simulink model "web_adc"  (Simulink 7.3)
settings: Solver=FixedStepDiscrete  SolverMode=SingleTasking  StartTime=0.0  StopTime=10.0  RelTol=1e-3
PreLoadFcn:
  | waijung.modelPreload; % Required for working with Waijung Blockset. Do not remove.
undefined symbols (not defined in the file): A0, A1, A2, A3, A7, B0, B1, B10, B11, B12, B13, C1, C2, C3, C4, C5, HSEOSC, Link, LQFP176, ST, STM32F417IG
libraries: simulink x4, waijung_webserver x3, stm32f4_io_lib x1, stm32f4_adc_lib x1, stm32f4_device_config_lib x1, amg_sqlite_dataserver x1
CloseFcn:
  | waijung.modelClose; % Required for working with Waijung Blockset. Do not remove.
settings Model: Creator=Krisada  LastModifiedBy=Krisada
settings OptimizationCC: OptimizeModelRefInitCode=on  LifeSpan=1
settings HardwareCC: ProdEndianess=LittleEndian  ProdHWDeviceType=ARM Compatible->Cortex - M4  TargetEndianess=LittleEndian  TargetHWDeviceType=ARM Compatible->Cortex - M4
settings RTWCC: SystemTargetFile=stm32f4.tlc  GenerateMakefile=off  TemplateMakefile=ert_default_tmf  Description=STM32F4 Target  ProcessScript=stm32f4_make_rtw_hook
settings CodeAppCC: IgnoreCustomStorageClasses=off
settings STFCustomTargetCC: ModelReferenceCompliant=off  CombineOutputUpdateFcns=on  ERTCustomFileBanners=on  SupportContinuousTime=off  SupportNonInlinedSFcns=off  SystemTargetFile=stm32f4.tlc
settings ERTTargetCC: MultiwordLength=2048  ModelReferenceCompliant=off  ParMdlRefBuildCompliant=off  CompOptLevelCompliant=off  ERTFirstTimeCompliant=off  ModelStepFunctionPrototypeControlCompliant=off  CPPClassGenCompliant=off  ExtModeMexFile=noextcomm  InlinedParameterPlacement=NonHierarchical  ERTSrcFileBannerTemplate=stm32f4_code_template.cgt  ERTHdrFileBannerTemplate=stm32f4_code_template.cgt  ERTDataSrcFileTemplate=stm32f4_code_template.cgt  ERTDataHdrFileTemplate=stm32f4_code_template.cgt  ERTCustomFileTemplate=stm32f4_file_process.tlc

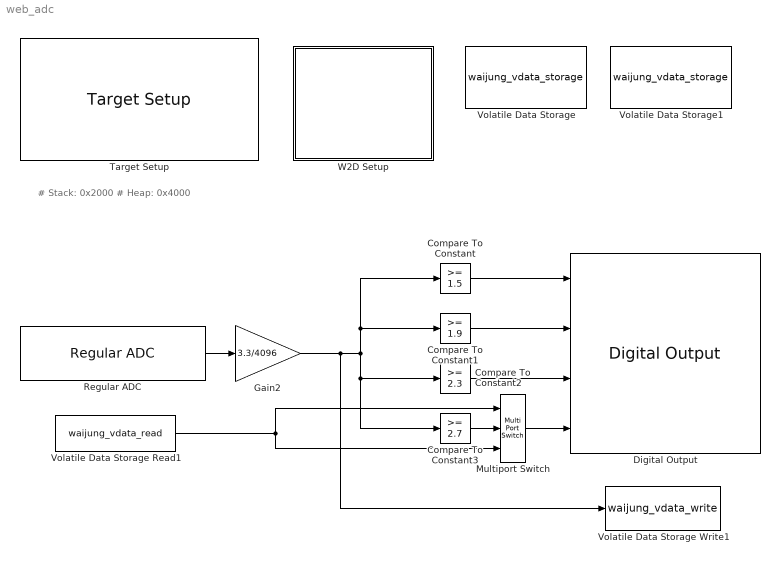
== system web_adc ==
  note: # Stack: 0x2000
      | # Heap: 0x4000
  Compare To Constant : simulink/Logic and Bit Operations/Compare To Constant  SystemSampleTime=-1  relop=>=  const=1.5  LogicOutDataTypeMode=uint8  ZeroCross=off
  Compare To Constant1 : simulink/Logic and Bit Operations/Compare To Constant  SystemSampleTime=-1  relop=>=  const=1.9  LogicOutDataTypeMode=uint8  ZeroCross=off
  Compare To Constant2 : simulink/Logic and Bit Operations/Compare To Constant  SystemSampleTime=-1  relop=>=  const=2.3  LogicOutDataTypeMode=uint8  ZeroCross=off
  Compare To Constant3 : simulink/Logic and Bit Operations/Compare To Constant  SystemSampleTime=-1  relop=>=  const=2.7  LogicOutDataTypeMode=uint8  ZeroCross=off
  Digital Output : stm32f4_io_lib/Digital Output  use_bitband=on  port=D  speed=100  porttype=Push Pull  porttypestr=PP  use_pin0=off  use_pin1=off  use_pin2=off  use_pin3=off  use_pin4=off  use_pin5=off  use_pin6=off  use_pin7=off  use_pin8=off  use_pin9=off  use_pin10=off  use_pin11=off  use_pin12=on  use_pin13=on  use_pin14=on  use_pin15=on  pinstr=GPIO_Pin_12 | GPIO_Pin_13 | GPIO_Pin_14 | GPIO_Pin_15  usedpinarray="[0  0  0  0  0  0  0  0  0  0  0  0  1  1  1  1]"  bitbandingstr=|  sampletime=-1  sampletimestr=0.01  blockid=DigitalOutput  enablecustomportlabel=off  globalinit=off  cinputportlabel=In1, In2  coutputportlabel=0
      | #define DigitalOutput_D12 Peripheral_BB(GPIOD->ODR, 12)  /* Output pin */
      | #define DigitalOutput_D13 Peripheral_BB(GPIOD->ODR, 13)  /* Output pin */
      | #define DigitalOutput_D14 Peripheral_BB(GPIOD->ODR, 14)  /* Output pin */
      | #define DigitalOutput_D15 Peripheral_BB(GPIOD->ODR, 15)  /* Output pin */
  Gain2 : Gain  Gain=3.3/4096  ParameterDataTypeMode=single  ParameterDataType=fixdt(1, 16)  ParameterScaling=2^0  ParamDataTypeStr=single  OutDataTypeMode=single  OutDataType=fixdt(1, 16)  OutScaling=2^0  OutDataTypeStr=single
  Multiport Switch : MultiPortSwitch  Inputs=2  zeroidx=on  OutDataType=fixdt(1, 16)  OutScaling=2^0
  Regular ADC : stm32f4_adc_lib/Regular ADC  adcmodule=1  outputdatatype=Double  prescaler=2  prescalerstr=ADC_Prescaler_Div2  chsamplingtime=Auto  chsamplingtimestr=ADC_SampleTime_480Cycles  read_an0=off  read_an1=off  read_an2=off  read_an3=off  read_an4=off  read_an5=off  read_an6=off  read_an7=off  read_an8=off  read_an9=off  read_an10=on  read_an11=off  read_an12=off  read_an13=off  read_an14=off  read_an15=off  read_an16=off  read_an17=off  read_an18=off  pinstr=GPIO_Pin_10  usedpinarray="[0  0  0  0  0  0  0  0  0  0  1  0  0  0  0  0  0  0  0]"  usedportidarray=[2]  usedpinidarray=[0]  usedpinidcount=1  sampletime=.01  blockid=RegularADC  enablecustomportlabel=off  cinputportlabel=0  coutputportlabel=Out1, Out2
  Target Setup : stm32f4_device_config_lib/Target Setup  Priority=100  compiler=GNU ARM  previous_compiler=GNU ARM  mcu=STM32F417IG (LQFP176)  mcustr=STM32F417IG  clockconfig=HSEOSC-8MHz  system_stm32f4xx_c_path=F:\trunk\targets\stm32f4_target\stm32f4\utils\system_stm32f4xx_default\STM32F40_41xxx\hseosc8mhz  showmemoryconfiguration=on  stacksize=0x2000  heapsize=0x4000  enableautocompiledownload=on  fullchiperase=off  programmerinterface=ST-Link  editctrlstr=on  compilercontrolstr=$(patsubst %, -I%, .) -mcpu=cortex-m4 -mthumb -mthumb-interwork -mfloat-abi=hard -mfpu=fpv4-sp-d16 -ffast-math -Wall -Wextra -Ofast  assemblercontrolstr=$(patsubst %, -I%, .) -mcpu=cortex-m4 -mthumb -mthumb-interwork -mfloat-abi=hard -mfpu=fpv4-sp-d16 -ffast-math -Wall -Wextra -Ofast -Wa,-amhls=$(<:.s=.lst) -D__STACK_SIZE=$(STACK_SIZE) -D__HEAP_SIZE=$(HEAP_SIZE)  linkercontrolstr=-T$(LD_SCRIPT) -g -Wl,-Map=$(MAP),--cref,--no-warn-mismatch -mcpu=cortex-m4 -mthumb -mthumb-interwork -mfloat-abi=hard -mfpu=fpv4-sp-d16 -specs=nosys.specs  runafterdownload=on  execprofile=None  profileruart=1  profilerbaud=115200  profilertxpin=D8  profilerinitstr=0.001,168000000,168000,115200,0  manualsetsampletime=off  sampletime=0.001  blockid=TargetSetup  systickreloadvalue=168000  hseval=8000000  lastprofileruart=1  hclk=168000000  flashorigin=0x8000000  flashlength=1024k  ramorigin=0x20000000  ramlength=128k  useextram=off
  Volatile Data Storage : S-Function  FunctionName=waijung_vdata_storage  Parameters=storagetype,storagename,initval,varname,buffersize,initvalstring,sampletime,sampletimestr,blockid,storagetypestr  EnableBusSupport=off  mask(waijung_vdata_storage){storagetype=single, storagename=adc, initval=0, varname=VolatileDataStorage_adc, buffersize=64, initvalstring='Initial string', webintegration=ReadOnly with KeyValuePair, weboutputformat='%f', webcgicallback=(void*)0, laststoragetype=single, sampletime=-1, sampletimestr=0.001, blockid=VolatileDataStorage, storagetypestr=float}
      mask prompts: storagetype "Storage Type"; storagename "Storage Name (must be a valid variable name)"; initval "Initial value (Apply at Power on Reset only)"; varname "Variable name"; buffersize "Size (bytes)"; initvalstring "Initial value (Apply at Power on Reset only)"; webintegration "Web CGI varget/varset integration"; weboutputformat "Web CGI varget output format"; webcgicallback "Web CGI varset callback"; laststoragetype "Last selected Storage Type"; sampletime "Sample time (sec)"; sampletimestr "Compiled sample time (sec) in string"; storagetypestr "Type string"
      mask help:
      | This block implements a volatile Data Storage.
      |
      | Web CGI varset/varget integratiopn:
      | Enable - In webserver application, allow remote access via http.
      | Disable - Variable is use in local only.
      mask init:
      | waijung_vdata_storage_callback('init');
      mask Help: web(fullfile(waijungdocroot,'Volatile_Data_Storage.htm'))
      mask StyleString: popup(double|single|uint32|int32|uint16|int16|uint8|int8|string),edit,edit,edit,edit,edit,popup(Disable|ReadOnly|Write/ Read|ReadOnly with KeyValuePair|Write/ Read with KeyValuePair),edit,edit,popup(double|single|uint32|int32|uint16|int16|uint8|int8|string),edit,edit,edit,edit
      mask CallbackString: waijung_vdata_storage_callback('storagetype');|waijung_vdata_storage_callback('storagename');|waijung_vdata_storage_callback('initval');|waijung_vdata_storage_callback('varname');||waijung_vdata_storage_callback('initvalstring');|waijung_vdata_storage_callback('webintegration');|waijung_vdata_storage_callback('weboutputformat');|||waijung_vdata_storage_callback('sampletime');|waijung_vdata_storage_callback('sampletimestr');|waijung_vdata_storage_callback('blockid');|
      mask Display: text(0.5, 0.5, 'Name: adc\nType: single','ver','middle','hor','center')
  Volatile Data Storage Read1 : S-Function  FunctionName=waijung_vdata_read  Parameters=storagename,varname,sampletime,sampletimestr,blockid,storagetype,storagetypestr  EnableBusSupport=off  mask(waijung_vdata_read){storagename=switch, varname=VolatileDataStorage1_switch, sampletime=inf, sampletimestr=0.01, blockid=VolatileDataStorageRead1, storagetype=uint8, storagetypestr=uint8_t}
      mask prompts: storagename "Storage Name"; varname "Variable name"; sampletime "Sample time (sec)"; sampletimestr "Compiled sample time (sec) in string"; storagetype "Data type"; storagetypestr "Data type string"
      mask help: This block implements read data from a buffer.
      mask init:
      | waijung_vdata_read_callback('init');
      mask Help: web(fullfile(waijungdocroot,'waijung_vdata_read.htm'))
      mask StyleString: popup(adc|switch),edit,edit,edit,edit,edit,edit
      mask CallbackString: waijung_vdata_read_callback('storagename');|waijung_vdata_read_callback('varname');|waijung_vdata_read_callback('sampletime');|waijung_vdata_read_callback('sampletimestr');|waijung_vdata_read_callback('blockid');|waijung_vdata_read_callback('storagetype');|
      mask Display: text(0.05, 0.5, 'Buffer: switch','ver','middle','hor','left');port_label('output',1,'D1(uint8)')
  Volatile Data Storage Write1 : S-Function  FunctionName=waijung_vdata_write  Parameters=storagename,varname,sampletime,sampletimestr,blockid,storagetype,storagetypestr  EnableBusSupport=off  mask(waijung_vdata_write){storagename=adc, varname=VolatileDataStorage_adc, sampletime=-1, sampletimestr=0.01, blockid=VolatileDataStorageWrite1, storagetype=single, storagetypestr=float}
      mask prompts: storagename "Storage Name"; varname "Variable name"; sampletime "Sample time (sec)"; sampletimestr "Compiled sample time (sec) in string"; storagetype "Data type"; storagetypestr "Data type string"
      mask help: This block implements write data to a buffer.
      mask init:
      | waijung_vdata_write_callback('init');
      mask Help: web(fullfile(waijungdocroot,'waijung_vdata_write.htm'))
      mask StyleString: popup(adc|switch),edit,edit,edit,edit,edit,edit
      mask CallbackString: waijung_vdata_write_callback('storagename');|waijung_vdata_write_callback('varname');|waijung_vdata_write_callback('sampletime');|waijung_vdata_write_callback('sampletimestr');|waijung_vdata_write_callback('blockid');|waijung_vdata_write_callback('storagetype');|
      mask Display: text(0.95, 0.5, 'Buffer: adc','ver','middle','hor','right');port_label('input',1,'D1(single)')
  Volatile Data Storage1 : S-Function  FunctionName=waijung_vdata_storage  Parameters=storagetype,storagename,initval,varname,buffersize,initvalstring,sampletime,sampletimestr,blockid,storagetypestr  EnableBusSupport=off  mask(waijung_vdata_storage){storagetype=uint8, storagename=switch, initval=0, varname=VolatileDataStorage1_switch, buffersize=64, initvalstring='Initial string', webintegration=Write/ Read with KeyValuePair, weboutputformat='%u', webcgicallback=(void*)0, laststoragetype=uint8, sampletime=-1, sampletimestr=0.001, blockid=VolatileDataStorage1, storagetypestr=uint8_t}
      mask prompts: storagetype "Storage Type"; storagename "Storage Name (must be a valid variable name)"; initval "Initial value (Apply at Power on Reset only)"; varname "Variable name"; buffersize "Size (bytes)"; initvalstring "Initial value (Apply at Power on Reset only)"; webintegration "Web CGI varget/varset integration"; weboutputformat "Web CGI varget output format"; webcgicallback "Web CGI varset callback"; laststoragetype "Last selected Storage Type"; sampletime "Sample time (sec)"; sampletimestr "Compiled sample time (sec) in string"; storagetypestr "Type string"
      mask help:
      | This block implements a volatile Data Storage.
      |
      | Web CGI varset/varget integratiopn:
      | Enable - In webserver application, allow remote access via http.
      | Disable - Variable is use in local only.
      mask init:
      | waijung_vdata_storage_callback('init');
      mask Help: web(fullfile(waijungdocroot,'Volatile_Data_Storage.htm'))
      mask StyleString: popup(double|single|uint32|int32|uint16|int16|uint8|int8|string),edit,edit,edit,edit,edit,popup(Disable|ReadOnly|Write/ Read|ReadOnly with KeyValuePair|Write/ Read with KeyValuePair),edit,edit,popup(double|single|uint32|int32|uint16|int16|uint8|int8|string),edit,edit,edit,edit
      mask CallbackString: waijung_vdata_storage_callback('storagetype');|waijung_vdata_storage_callback('storagename');|waijung_vdata_storage_callback('initval');|waijung_vdata_storage_callback('varname');||waijung_vdata_storage_callback('initvalstring');|waijung_vdata_storage_callback('webintegration');|waijung_vdata_storage_callback('weboutputformat');|||waijung_vdata_storage_callback('sampletime');|waijung_vdata_storage_callback('sampletimestr');|waijung_vdata_storage_callback('blockid');|
      mask Display: text(0.5, 0.5, 'Name: switch\nType: uint8','ver','middle','hor','center')
  W2D Setup : Subsystem
  wires:
  Regular ADC/1 -> Gain2/1
  Compare To Constant/1 -> Digital Output/1
  Compare To Constant1/1 -> Digital Output/2
  Compare To Constant2/1 -> Digital Output/3
  Gain2/1 -> Compare To Constant1/1, Compare To Constant/1, Compare To Constant2/1, Compare To Constant3/1, Volatile Data Storage Write1/1
  Multiport Switch/1 -> Digital Output/4
  Volatile Data Storage Read1/1 -> Multiport Switch/1, Multiport Switch/3
  Compare To Constant3/1 -> Multiport Switch/2

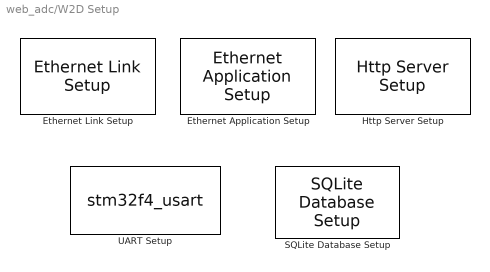
== system web_adc/W2D Setup ==
  Ethernet Application Setup : waijung_webserver/Ethernet Application Setup  conf=Setup  ipaddress=192.168.1.30  netmask=255.255.255.0  gateway=192.168.1.1  macaddress=02-00-00-00-00-00  dhcp=off  timerscaler=10  portpinstr=0  sampletime=0.001  blockid=W2DSetupEthernetApplicationSetup  inputporttype=[]  inputportwidth=[]  inputportlabel={}  outputporttype=[]  outputportwidth=[]  outputportlabel={}  compat=0  optionstring="[\"Dummy\",\"192\",\"168\",\"1\",\"30\",\"255\",\"255\",\"255\",\"0\",\"192\",\"168\",\"1\",\"1\",\"02\",\"00\",\"00\",\"00\",\"00\",\"00\",\"off\",\"10\"]"
  Ethernet Link Setup : waijung_webserver/Ethernet Link Setup  conf=Setup  interfacepin=Profile #1  wj_interfacetype=MII  pin_mdio=A2  pin_mdc=C1  pin_pps=Not used  pin_crs=A0  pin_col=A3  pin_dv=A7  pin_rxclk=A1  pin_rxer=B10  pin_rxd0=C4  pin_rxd1=C5  pin_rxd2=B0  pin_rxd3=B1  pin_txclk=C3  pin_txen=B11  pin_txd0=B12  pin_txd1=B13  pin_txd2=C2  pin_txd3=E2  portpinstr=A0,A1,A2,A3,A7,B0,B1,E2,B10,B11,B12,B13,C1,C2,C3,C4,C5  sampletime=inf  blockid=W2DSetupEthernetLinkSetup  inputporttype=[]  inputportwidth=[]  inputportlabel={}  outputporttype=[]  outputportwidth=[]  outputportlabel={}  compat=0  optionstring="[\"xxx\",\"on\",\"on\",\"on\",\"off\",\"on\",\"off\",\"off\",\"off\",\"off\",\"on\",\"on\",\"on\",\"on\",\"on\",\"on\",\"on\",\"off\",\"on\",\"on\",\"on\",\"on\",\"on\",\"on\",\"on\",\"on\",\"on\",\"on\",\"A\",\"0\",\"A\",\"1\",\"A\",\"2\",\"A\",\"3\",\"A\",\"7\",\"B\",\"0\",\"B\",\"1\",\"N\",\"ot used\",\"E\",\"2\",\"B\",\"10\",\"B\",\"11\",\"B\",\"12\",\"B\",\"13\",\"C\",\"1\",\"C\",\"2\",\"C\",\"3\",\"C\",\"4\",\"C\",\"5\",\"MII\"]"
  Http Server Setup : waijung_webserver/Http Server Setup  conf=Setup  port=80  ssl=Disable  sqlite=Enable  iap=Disable  mempool=8  debugport=Disable  portpinstr=0  sampletime=inf  blockid=W2DSetupHttpServerSetup  inputporttype=[]  inputportwidth=[]  inputportlabel={}  outputporttype=[]  outputportwidth=[]  outputportlabel={}  compat=0  optionstring="[\"80\",\"0\",\"0\",\"Enable\",\"Disable\",\"8\",\"17.02a\",\"\",\"\",\"\",\"adc\",\"single\",\"VolatileDataStorage_adc\",\"1\",\"0\",\"1\",\"(void*)0\",\"%f\",\"\",\"\",\"switch\",\"uint8\",\"VolatileDataStorage1_switch\",\"1\",\"1\",\"1\",\"(void*)0\",\"%u\",\"\",\"\"]"
  SQLite Database Setup : amg_sqlite_dataserver/SQLite Database Setup  Priority=1  port=UART6  timeout=5  buffersize=8192  reset=Software  resetport=A  resetpin=0  inputtypearray=[0]  outputtypearray=[0]  sampletime=inf  sampletimestr=0.001  blockid=W2DSetupSQLiteDatabaseSetup
  UART Setup : S-Function  Priority=1  FunctionName=stm32f4_usart  Parameters=configuration,uartmodule,transfer,baudrate,inputtype,outputtype,confstr,binheaderarray,binterminatorarray,asciiheader,asciiterminator,bindatalength,packetmode,varname,sampletime,sampletimestr,blockid  EnableBusSupport=off  mask(stm32f4_usart){configuration=Setup, uartmodule=6, baudrate=1e6, databits=8, parity=No, stopbit=1, remaptxpin=C6, remaprxpin=C7, flowcontrol=None, remapctspin=Not used, remaprtspin=Not used, advanceoptions=on, rxbuffersize=2048, txbuffersize=1024, transfer=Blocking, packetmode=Ascii, binheader='7E 7E', binterminator='03 03', porttype_double=1, porttype_single=0, porttype_int8=1, porttype_uint8=0, porttype_int16=0, porttype_uint16=0, porttype_int32=0, porttype_uint32=0, asciiformat='%d,%f', rx_asciiterminator=CRLF (0x0D 0x0A - "\r\n"), tx_asciiterminator=CR (0x0D - "\r"), storagename=<empty>, varname=, inputtype=[0], outputtype=[0], binheaderarray=[0], binterminatorarray=[0], bindatalength=0, asciiheader='', asciiterminator=[0], sampletime=-1, sampletimestr=0.001, blockid=W2DSetupUARTSetup, confstr=[ "dummy", "1", "C", "6", "1", "C", "7", "0", "*", "*", "0", "*", "*", "2", "5", "6", "2", "5", "1", "1024", "2048", "2", "6", "1e6", "8", "No", "1", "None", "USART6"], lastmodule=6}
      mask prompts: uartmodule "UART Module"; baudrate "Baud rate (bps)"; databits "Data bits"; stopbit "Stop bit"; remaptxpin "Tx Pin"; remaprxpin "Rx Pin"; flowcontrol "Hardware flow control"; remapctspin "HW Flow control, CTS Pin"; remaprtspin "HW Flow control, RTS Pin"; advanceoptions "Advance options"; rxbuffersize "Rx buffer size (bytes)"; txbuffersize "Tx buffer size (bytes)"; packetmode "Packet mode"; binheader "Binary header (example: '7E 7E')"; binterminator "Binary terminator (example: '03 03')"; porttype_double "Number of data port, type DOUBLE"; porttype_single "Number of data port, type SINGLE"; porttype_int8 "Number of data port, type INT8"; porttype_uint8 "Number of data port, type UINT8"; porttype_int16 "Number of data port, type INT16"; porttype_uint16 "Number of data port, type UINT16"; porttype_int32 "Number of data port, type INT32"; porttype_uint32 "Number of data port, type UINT32"; asciiformat "Ascii format"; rx_asciiterminator "End of packet"; tx_asciiterminator "End of packet"; storagename "Buffer"; varname "Var name"; inputtype "Input data type"; outputtype "Output data type"; binheaderarray "Binary header"; binterminatorarray "Binary terminator"; bindatalength "Binary data length"; asciiheader "Ascii header (printf format)"; asciiterminator "Ascii terminator"; sampletime "Sample time (sec)"; sampletimestr "Compiled sample time (sec) in string"; confstr "Configuration string"; lastmodule "Last module selected"
      mask init:
      | stm32f4_usart_callback('init');
      mask Help: web(fullfile(waijungdocroot,'stm32f4_usart_setup.htm'), '-browser')
      mask StyleString: popup(Setup|Tx|Rx),popup(1|2|3|4|5|6),edit,popup(8),popup(No|Odd|Even),popup(0.5|1|1.5|2),popup(Not used|C6|G14),popup(Not used|C7|G9),popup(None|RTS|CTS|RTS/CTS),popup(Not used|G13|G15),popup(Not used|G8|G12),checkbox,popup(16|32|64|128|256|512|1024|2048),popup(16|32|64|128|256|512|1024|2048),popup(Blocking|Non-Blocking),popup(Ascii|Binary|String Buffer),edit,edit,edit,edit,edit,edit,edit,edit,edit,edit,edit,popup(CR (0x0D - "\r")|LF (0x0A - "\n")|CRLF (0x0D 0x0A - "\r\n")),popup(CR (0x0D - "\r")|LF (0x0A - "\n")|CRLF (0x0D 0x0A - "\r\n")|None),popup(<empty>),edit,edit,edit,edit,edit,edit,edit,edit,edit,edit,edit,edit,edit
      mask CallbackString: stm32f4_usart_callback('configuration');|stm32f4_usart_callback('uartmodule');|stm32f4_usart_callback('baudrate');||||||stm32f4_usart_callback('flowcontrol');|||stm32f4_usart_callback('advanceoptions');|||stm32f4_usart_callback('transfer');|stm32f4_usart_callback('packetmode');|stm32f4_usart_callback('binheader');|stm32f4_usart_callback('binterminator');|stm32f4_usart_callback('porttype');|stm32f4_usart_callback('porttype');|stm32f4_usart_callback('porttype');|stm32f4_usart_callback('porttype');|stm32f4_usart_callback('porttype');|stm32f4_usart_callback('porttype');|stm32f4_usart_callback('porttype');|stm32f4_usart_callback('porttype');|stm32f4_usart_callback('asciiformat');|stm32f4_usart_callback('rx_asciiterminator');|stm32f4_usart_callback('tx_asciiterminator');|stm32f4_usart_callback('storagename');|stm32f4_usart_callback('varname');||||||||stm32f4_usart_callback('sampletime');|stm32f4_usart_callback('sampletimestr');|stm32f4_usart_callback('blockid');||
      mask Display: text(0.5, 0.5, 'Module: USART6_Setup\nBaud (Bps): 1e6\nDMA Buffer: 1024/2048\nTx/Rx Pin: C6/C7','ver','middle','hor','center');
